simulink model "mod_sim_VTMS"  (R2018b)
settings: Solver=FixedStepDiscrete  StartTime=0.0  StopTime=t_Simulation  FixedStep=delta_t  RelTol=1e-3
values from neighbouring files (symbols this model uses):
  P_charge = 150    [main_sim_VTMS.m]
undefined symbols (not defined in the file or in its folder): A_EMaschine_Getriebe, A_j_c, A_Stirn, Anzahl_Peltierelemente, b_Batteriepack, b_c, b_EMaschine, b_Getriebe, b_j, b_Ladegeraet, BatPara, c_W, delta_t, DiscIntNeverNeededParam, e_Fahrzeug, eta_EMaschine_Break_M_EMaschine, eta_EMaschine_Break_n_EMaschine, eta_EMaschine_Faktor_Volllast, eta_EMaschine_Table, eta_Getriebe, eta_Ladegeraet, eta_Leistungselektronik_Break_M_EMaschine, eta_Leistungselektronik_Break_n_EMaschine, eta_Leistungselektronik_Faktor_Volllast, eta_Leistungselektronik_Table, f_R, I_DT_U_Break_DT, I_DT_U_Break_U, I_DT_U_Value_I, i_Getriebe, I_max, Ladevorgang, M_EMaschine_max, m_Fahrzeug, m_Zuladung, n_Zelle, P_Nebenverbraucher, p_Zelle, Peltier_Max_Eff, Q_DT_U_Break_DT, Q_DT_U_Break_U, Q_DT_U_Value_Q, Q_Imax_DT_Break_DT, Q_Imax_DT_Value_Q, r_dynamisch, rho_Luft, s_Zelle, SOC_init, Steuerung_Kuehlerluefter, Steuerung_Pumpe, Steuerung_Ventil, switch_BP_Zyklus, T_Batteriepack_init, T_EMaschine_Getriebe_init, T_Ladegeraet_init, T_Ladegeraet_Offset, T_Leistungselektronik_init, T_Offset_Batteriepack, T_Offset_EMaschine_Getriebe, T_Offset_Leistungselektronik ... (+36)
libraries: simulink x3, simulink_extras x2
(part 3 of 5)

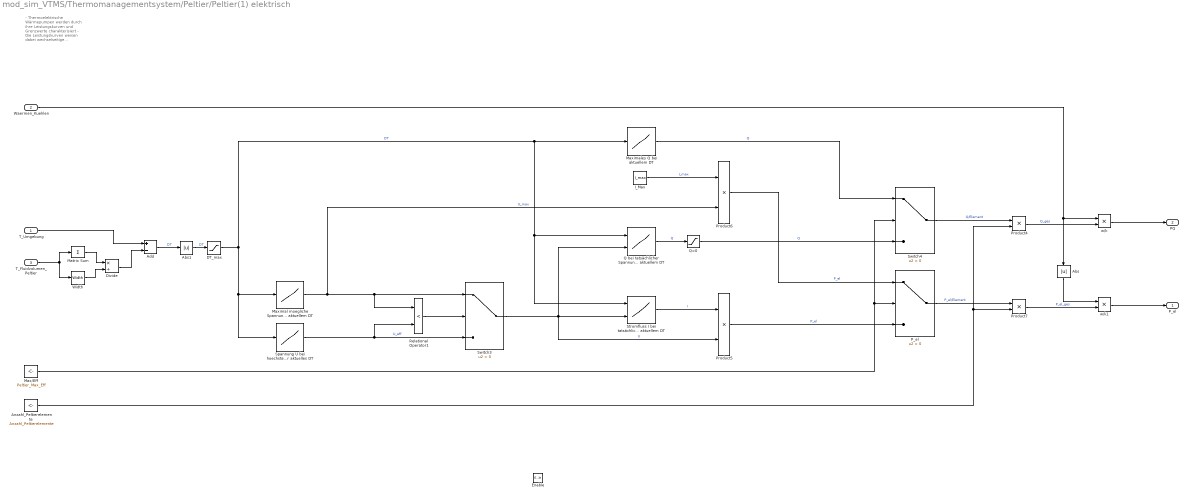
== system mod_sim_VTMS/Thermomanagementsystem/Peltier/Peltier(1) elektrisch ==
  note: - Thermoelektrische Wärmepumpen werden durch ihre Leistungskurven und Grenzwerte charakterisiert
      | - Die Leistungskurven weisen dabei wechselseitige Abhängigkeiten von der Temperaturdifferenz zwischen heißer und kalter Seite, der anliegenden Spannung, dem Strom und dem Wärmestrom auf.
      | - Für die Parameter existieren dabei Maximalwerte, die die Leistung und den Wärmefluss limitieren.
      | - Die Leistungskurven in diesem Modell sind aus dem Datenblatt einer beispielhaften Wärmepumpe entnommen.
      |
      | - Das Modell des Peltier-Elements hat keine eigene Masse und weist folglich keine eigene Temperatur auf
      | - Der resultierende Wärmestrom wird gesamthaft von einer Seite zur anderen transportiert, ohne dabei die Komponente aufzuheizen. Dadurch wirkt ein Wärmestrom direkt zwischen Umgebung und Kühlkreislauf und die Temperaturdifferenz zwischen heißer und kalter Seite ergibt sich aus der Umgebungstemperatur und der Temperatur des Kühlfluids
      | - Tendenziell ergibt sich für niedrigere Wärmeleistungen ein höherer COP. Deswegen wurden im Modell der Wärmepumpe zwei Betriebsmodi eingefügt, ein effektiver Modus und ein Leistungsmodus.
      | - Der Betriebsmodus wird über das Signal Max_Eff gesteuert, das den Wert 1 für maximale Leistung und den Wert -1 für maximale Effizienz annimmt.
      |
      | - Im effizienten Modus wird die Spannung an der Komponente so geregelt, dass sich für die aktuelle Temperaturdifferenz die höchste Leistungszahl ergibt. Das Maximum des COP liegt bei niedrigen Spannungen vor. Deswegen ergeben sich in diesem Zustand trotz der hohen Leistungszahl nur niedrige Wärmeleistungen.
      | - Im Leistungsmodus wird immer der maximal mögliche Wärmestrom erzeugt, ungeachtet vom COP. Dafür wird die Spannung so geregelt, dass sich entsprechend der aktuellen Temperaturdifferenz der maximale Strom einstellt, dieser aber nicht überschritten wird.
      |
      | Für detaillierte Informationen wird auf die schriftliche Arbeit von Bernhardt "Entwicklung und Auslegung eines innovativen Thermomanagementsystems für Elektrofahrzeuge" verwiesen.
  T_Umgebung : Inport
  Waermen_Kuehlen : Inport  Port=2
  T_Fluidvolumen_Peltier : Inport  Port=3
  Enable : EnablePort
  Abs : Abs
  Abs1 : Abs
  Add : Sum  Inputs=+-
  Anzahl_Peltierelemente : Constant  Value=Anzahl_Peltierelemente
  DT_max : Saturate  UpperLimit=60  LowerLimit=0
  Divide : Product  Inputs=*/
  I_Max : Constant  Value=I_max
  Matrix Sum : Sum  Inputs=+
  Max/Eff : Constant  Value=Peltier_Max_Eff
  Maximal moegliche Spannung bei aktuellem DT : Lookup_n-D  NumberOfTableDimensions=1  BreakpointsForDimension1=U_max_Break_DT  BreakpointsForDimension2=[1:3]  Table=U_max_Value_U  InternalRulePriority=Speed  RndMeth=Simplest  InputSameDT=on
  Maximales Q bei aktuellem DT : Lookup_n-D  NumberOfTableDimensions=1  BreakpointsForDimension1=Q_Imax_DT_Break_DT  BreakpointsForDimension2=[1:3]  Table=Q_Imax_DT_Value_Q  InternalRulePriority=Speed  RndMeth=Simplest  InputSameDT=on
  P_el : Switch  Criteria=u2 > Threshold
  Product{4..7} (4 alike) : Product
  Q bei tatsächlicher Spannung U und aktuellem DT : Lookup_n-D  BreakpointsForDimension1=Q_DT_U_Break_DT  BreakpointsForDimension2=Q_DT_U_Break_U  Table=Q_DT_U_Value_Q  InternalRulePriority=Speed  RndMeth=Simplest  InputSameDT=on
  Q>0 : Saturate  UpperLimit=inf  LowerLimit=0
  Relational Operator1 : RelationalOperator  Operator=<  OutDataTypeStr=boolean  RndMeth=Simplest
  Spannung U bei hoechsten COP fuer aktuelles DT : Lookup_n-D  NumberOfTableDimensions=1  BreakpointsForDimension1=U_COP_max_Break_DT  BreakpointsForDimension2=[1:3]  Table=U_COP_max_Value_U  InternalRulePriority=Speed  RndMeth=Simplest  InputSameDT=on
  Stromfluss I bei tatsächlicher Spannung U und aktuellem DT : Lookup_n-D  BreakpointsForDimension1=I_DT_U_Break_DT  BreakpointsForDimension2=I_DT_U_Break_U  Table=I_DT_U_Value_I  InternalRulePriority=Speed  RndMeth=Simplest  InputSameDT=on
  Switch3 : Switch  Criteria=u2 > Threshold
  Switch4 : Switch  Criteria=u2 > Threshold
  Width : Width
  w/k : Product
  w/k1 : Product
  "P_el " : Outport
  PQ : Outport  Port=2
  wires:
  Waermen_Kuehlen/1 -> Abs/1, w/k/1
  Relational Operator1/1 -> Switch3/2
  Q bei tatsächlicher Spannung U und aktuellem DT/1 -> Q>0/1  "Q"
  Maximal moegliche Spannung bei aktuellem DT/1 -> Product6/2, Switch3/1, Relational Operator1/1  "U_max"
  DT_max/1 -> Stromfluss I bei tatsächlicher Spannung U und aktuellem DT/1, Q bei tatsächlicher Spannung U und aktuellem DT/1, Maximales Q bei aktuellem DT/1, Spannung U bei hoechsten COP fuer aktuelles DT/1, Maximal moegliche Spannung bei aktuellem DT/1  "DT"
  Add/1 -> Abs1/1  "DT"
  Switch3/1 -> Q bei tatsächlicher Spannung U und aktuellem DT/2, Product5/2, Stromfluss I bei tatsächlicher Spannung U und aktuellem DT/2  "U"
  P_el/1 -> Product7/1  "P_el/Element"
  Product6/1 -> P_el/1  "P_el"
  I_Max/1 -> Product6/1  "I_max"
  Product4/1 -> w/k/2  "Q_ges"
  Spannung U bei hoechsten COP fuer aktuelles DT/1 -> Switch3/3, Relational Operator1/2  "U_eff"
  Max/Eff/1 -> Switch4/2, P_el/2
  Switch4/1 -> Product4/1  "Q/Element"
  w/k/1 -> PQ/1
  Stromfluss I bei tatsächlicher Spannung U und aktuellem DT/1 -> Product5/1  "I"
  Product5/1 -> P_el/3  "P_el"
  Anzahl_Peltierelemente/1 -> Product4/2, Product7/2
  Abs1/1 -> DT_max/1  "DT"
  Maximales Q bei aktuellem DT/1 -> Switch4/1  "Q"
  Product7/1 -> w/k1/2  "P_el_ges"
  Divide/1 -> Add/2
  Width/1 -> Divide/2
  T_Umgebung/1 -> Add/1
  Matrix Sum/1 -> Divide/1
  T_Fluidvolumen_Peltier/1 -> Matrix Sum/1, Width/1
  Q>0/1 -> Switch4/3  "Q"
  w/k1/1 -> "P_el "/1
  Abs/1 -> w/k1/1

== system mod_sim_VTMS/Thermomanagementsystem/Peltier/Peltier(1) thermisch ==
  note: -> Das Peltier-Element selber hat keine Masse
      | -> Es besitzt dadurch keine eigene Temperatur
      |
      | -> Es Transportiert die komplette Leistung als Wärme- oder Kühlleistung in das Kuehlwasser
      | -> Dafür wird die Leistung durch die Anzahl an finiten Volumen geteilt
      |
      | -> Die Peltier-Leistung wird in Form eines Vektors der Größe des Temperaturvektors, also der Anzahl an finiten Volumen in der Fluidkomponente, übertragen.
      | -> Dafür wird ein Einsvektor der Größe erstellt und mit der Leistung pro fintem Volumen multipliziert
  P_Peltier [W] : Inport
  T_FinitesVolumen [K] : Inport  Port=2
  Divide : Product  Inputs=*/
  Divide1 : Product  Inputs=*/
  Divide2 : Product  Inputs=**
  Width : Width
  PQ_Peltier_FinitesVolumen [W] : Outport
  wires:
  Width/1 -> Divide/2
  Divide1/1 -> Divide2/2
  Divide/1 -> Divide2/1
  T_FinitesVolumen [K]/1 -> Divide1/2, Divide1/1, Width/1
  Divide2/1 -> PQ_Peltier_FinitesVolumen [W]/1
  P_Peltier [W]/1 -> Divide/1  "P_Peltier [W]"

== system mod_sim_VTMS/Thermomanagementsystem/Rad_Betriebspunkt/Abbruch, wenn v_Fahrzeug > Schwellwert ==
  v_Fahrzeug [m/s] : Inport
  Enable : EnablePort
  Abbruchgeschwindigkeit [km/h] : Constant  Value=v_end
  Gain4 : Gain  Gain=3.6
  Relational Operator : RelationalOperator  OutDataTypeStr=boolean  RndMeth=Simplest
  Stop Simulation : Stop
  wires:
  Gain4/1 -> Relational Operator/1
  Abbruchgeschwindigkeit [km/h]/1 -> Relational Operator/2
  Relational Operator/1 -> Stop Simulation/1
  v_Fahrzeug [m/s]/1 -> Gain4/1

== system mod_sim_VTMS/Thermomanagementsystem/Schlauch/Schlauch thermisch ==
  note: -> Ein Schlauch besitzt keine eigene Temperatur und wird als adiabat zu seiner Umgebung betrachtet
      | -> Es gibt also keinen Wärmeaustausch zwischen Umgebungsluft und Kühlflüssigkeit
      | -> Ein Schlauch besitzt zudem nur 1 Strömungsgebiet bzw. 1 Kühlflüssigkeit
      | -> Deshalb existiert bei einem Schlauch kein Wärmeaustausch zwischen der Kühlflüssigkeit im Strömungsgebiet und ihrer Umgebung
      | -> Deswegen wird T_FinitesVolumen_i mit 0 multipliziert, um PQ_Schlauch_FinitesVolumen_i = 0 zu erhalten
      | -> Mit den unbenutzten Größen PV_Kuehlfluessigkeit und v_Fahrzeug (für die Wärmeübertragungsfähigkeit) sowie T_Umgebung und T_FinitesVolumen (für die Temperaturdifferenz zwischen Umgebungsluft und Kühlflüssigkeit) könnte aber ein Wärmeaustausch zwischen Umgebungsluft und Kühlflüssigkeit nachträglich modelliert werden, falls dies gewünscht sein sollte
  T_FinitesVolumen [K] : Inport
  PV_Kuehlfluessigkeit [m^3*s^-1] : Inport  Port=2
  T_Umgebung [K] : Inport  Port=3
  v_Fahrzeug [m*s^-1] : Inport  Port=4
  Gain : Gain  Gain=0
  Terminator : Terminator
  Terminator1 : Terminator
  Terminator2 : Terminator
  PQ_Schlauch_FinitesVolumen [W] : Outport
  wires:
  Gain/1 -> PQ_Schlauch_FinitesVolumen [W]/1
  PV_Kuehlfluessigkeit [m^3*s^-1]/1 -> Terminator/1
  v_Fahrzeug [m*s^-1]/1 -> Terminator2/1
  T_Umgebung [K]/1 -> Terminator1/1
  T_FinitesVolumen [K]/1 -> Gain/1

== system mod_sim_VTMS/Thermomanagementsystem/Wärmetauscher/Waermetauscher thermisch ==
  note: Gleichstromwärmetauscher (Art_Waermetauscher = 1):
      | PQ_Waermetauscher(1)_FinitesVolumen_i = UA_Waermetauscher_FinitesVolumen * (T_FinitesVolumen(2)_i - T_FinitesVolumen(1)_i) für i = 1:n
      | PQ_Waermetauscher(2)_FinitesVolumen_i = UA_Waermetauscher_FinitesVolumen * (T_FinitesVolumen(1)_i - T_FinitesVolumen(2)_i) für i = 1:n
      |
      | Gegenstromwärmetauscher (Art_Waermetauscher = -1):
      | PQ_Waermetauscher(1)_FinitesVolumen_i = UA_Waermetauscher_FinitesVolumen * (T_FinitesVolumen(2)_n+1-i - T_FinitesVolumen(1)_i) für i = 1:n
      | PQ_Waermetauscher(2)_FinitesVolumen_i = UA_Waermetauscher_FinitesVolumen * (T_FinitesVolumen(1)_n+1-i - T_FinitesVolumen(2)_i) für i = 1:n
      |
      | mit UA_Waermetauscher_FinitesVolumen = f (PV_Kuehlfluessigkeit(1), PV_Kuehlfluessigkeit(2))
      |
      | -> UA_Waermetauscher_FinitesVolumen ist für jedes finite Volumen des 1. bzw. 2. Strömungsgebiets eines Wärmetauschers identisch, weil das 1. bzw. 2. Strömungsgebiet eines Wärmetauschers durch identische finite Volumen örtlich diskretisiert ist und weil im gesamten 1. bzw. 2. Strömungsgebiet eines Wärmetauschers der gleiche Volumenstrom der Kühlflüssigkeit vorliegt
      | -> Im Thermomanagementsystemmodell geht der Massenstrom bzw. Volumenstrom innerhalb einer Fluid_Komponente bei jeder Fluid_Komponente stets vom 1. finiten Volumen zum n. finiten Volumen
      | -> Bei einem Gleichstromwärmetauscher sind die Kühlflüssigkeitsströme in seinen zwei Strömungsgebieten gleich gerichtet
      | -> Deswegen tauscht das i. finite Volumen des einen Strömungsgebiets des Wärmetauschers mit dem i. finiten Volumen des anderen Strömungsgebiets des Wärmetauschers Wärme aus
      | -> Bei einem Gegenstromwärmetauscher sind die Kühlflüssigkeitsströme in seinen zwei Strömungsgebieten entgegengesetzt gerichtet
      | -> Deswegen tauscht das i. finite Volumen des einen Strömungsgebiets des Wärmetauschers mit dem n+1-i. finiten Volumen des anderen Strömungsgebiets des Wärmetauschers Wärme aus
  note: -> Ein Wärmetauscher besitzt keine eigene Temperatur und wird als adiabat zu seiner Umgebung betrachtet
      | -> Es gibt also keinen Wärmeaustausch zwischen Umgebungsluft und Kühlflüssigkeit, sondern nur einen Wärmeaustausch zwischen den beiden Kühlflüssigkeiten eines Wärmetauschers
      | -> Mit den unbenutzten Größen T_Umgebung (für die Temperaturdifferenz zwischen Umgebungsluft und Kühlflüssigkeit) und v_Fahrzeug (für die Wärmeübertragungsfähigkeit) könnte aber ein Wärmeaustausch zwischen Umgebungsluft und Kühlflüssigkeit nachträglich modelliert werden, falls dies gewünscht sein sollte
  T_FinitesVolumen(1) [K] : Inport
  PV_Kuehlfluessigkeit(1) [m^3*s^-1] : Inport  Port=2
  T_FinitesVolumen(2) [K] : Inport  Port=3
  PV_Kuehlfluessigkeit(2) [m^3*s^-1] : Inport  Port=4
  T_Umgebung [K] : Inport  Port=5
  v_Fahrzeug [m*s^-1] : Inport  Port=6
  Art_Waermetauscher : Constant  Value=0  VectorParams1D=off
  Flip : DSPFlip
  Flip1 : DSPFlip
  Product : Product
  Product1 : Product
  Subtract : Sum  Inputs=+-
  Subtract1 : Sum  Inputs=+-
  Switch : Switch  Criteria=u2 > Threshold
  Switch1 : Switch  Criteria=u2 > Threshold
  Terminator : Terminator
  Terminator1 : Terminator
  n-D Lookup Table : Lookup_n-D  BreakpointsForDimension1=0  BreakpointsForDimension2=0  BreakpointsForDimension3=[5, 7]  BeginIndexSearchUsingPreviousIndexResult=on  Table=0  ExtrapMethod=Clip  UseLastTableValue=on  InternalRulePriority=Speed  RndMeth=Simplest  InputSameDT=on
  PQ_Waermetauscher(1)_FinitesVolumen [W] : Outport
  PQ_Waermetauscher(2)_FinitesVolumen [W] : Outport  Port=2
  wires:
  PV_Kuehlfluessigkeit(1) [m^3*s^-1]/1 -> n-D Lookup Table/1
  Subtract/1 -> Product/2
  n-D Lookup Table/1 -> Product/1, Product1/1  "UA_Waermetauscher_FinitesVolumen [W*K^-1]"
  Product/1 -> PQ_Waermetauscher(1)_FinitesVolumen [W]/1
  v_Fahrzeug [m*s^-1]/1 -> Terminator1/1
  T_Umgebung [K]/1 -> Terminator/1
  PV_Kuehlfluessigkeit(2) [m^3*s^-1]/1 -> n-D Lookup Table/2
  Flip/1 -> Switch/3
  Switch/1 -> Subtract/1
  T_FinitesVolumen(2) [K]/1 -> Switch/1, Flip/1, Subtract1/2
  Art_Waermetauscher/1 -> Switch/2, Switch1/2
  Subtract1/1 -> Product1/2
  Switch1/1 -> Subtract1/1
  Flip1/1 -> Switch1/3
  T_FinitesVolumen(1) [K]/1 -> Subtract/2, Switch1/1, Flip1/1
  Product1/1 -> PQ_Waermetauscher(2)_FinitesVolumen [W]/1

== system mod_sim_VTMS/Thermomanagementsystem/Batteriepack/Batteriepack(1) elektrisch/Batteriepackgrößen ==
  note: P_Verlust_Batteriepack = (P_Verlust_Zelle_irreversibel + P_Verlust_Zelle_reversibel) * n_Zelle
  note: U_Batteriepack = U_Zelle * s_Zelle
  note: I_Batteriepack = I_Zelle * p_Zelle
  note: -> Da alle Zellen als komplett identisch angenommen werden, entspricht der Wirkungsgrad einer Zelle dem Wirkungsgrad des gesamten Batteriepacks
      |
      | eta_Batteriepack = eta_Zelle
      | = P_Zelle / (P_Zelle + P_Verlust_Zelle_irreversibel) für P > 0
      | = (P_Zelle + P_Verlust_Zelle_irreversibel) / P_Zelle für P < 0
      |
      | -> Die Berechnung wird nur ausgeführt, wenn P_Zelle ~= 0 ist, weil bei P_Zelle = 0 auch P_Verlust_Zelle_irreversibel = 0 ist und dadurch eine Berechnung mit Division durch 0 durchgeführt werden würde (P_Zelle kann im Fahrbetrieb nicht < 0 sein, weil von den Rädern an den Antriebsstrang keine negativen Leistungsanforderungen übertragen werden)
      | -> Während der Batterieladung wird diese mit einem P < 0 geladen
      | -> Dies wird über das Subsystem "Enabled Subsystem" realisiert
      | -> Wenn P_Zelle = 0 ist, wird die Berechnung nicht durchgeführt und eta_Batteriepack solange auf dem gleichen Wert gehalten, bis P_Zelle wieder ~= 0 ist
  note: -> Der SOC des Batteriepacks entspricht dem SOC einer Zelle, weil alle Zellen im Batteriepack den gleichen Wert aufweisen
      |
      | SOC_Batteriepack = SOC_Zelle
  P_Zelle [W] : Inport
  I_Zelle [A] : Inport  Port=2
  U_Zelle [V] : Inport  Port=3
  SOC_Zelle [-] : Inport  Port=4
  P_Verlust_Zelle_irreversibel [W] : Inport  Port=5
  P_Verlust_Zelle_reversibel [W] : Inport  Port=6
  Abs : Abs
  Add : Sum
  Constant : Constant  Value=p_Zelle  VectorParams1D=off
  Constant1 : Constant  Value=s_Zelle  VectorParams1D=off
  Constant2 : Constant  Value=n_Zelle  VectorParams1D=off
  Enabled Subsystem : Subsystem  TreatAsAtomicUnit=on
  Product : Product
  Product1 : Product
  Product2 : Product
  I_Batteriepack [A] : Outport
  U_Batteriepack [V] : Outport  Port=2
  "SOC_Batteriepack [-] " : Outport  Port=3
  eta_Batteriepack [%] : Outport  Port=4
  P_Verlust_Batteriepack [W] : Outport  Port=5
  wires:
  Constant/1 -> Product/2
  I_Zelle [A]/1 -> Product/1
  Product/1 -> I_Batteriepack [A]/1
  U_Zelle [V]/1 -> Product1/1
  Constant1/1 -> Product1/2
  Product1/1 -> U_Batteriepack [V]/1
  Constant2/1 -> Product2/2
  Product2/1 -> P_Verlust_Batteriepack [W]/1
  Add/1 -> Product2/1
  P_Verlust_Zelle_reversibel [W]/1 -> Add/1
  SOC_Zelle [-]/1 -> "SOC_Batteriepack [-] "/1
  P_Verlust_Zelle_irreversibel [W]/1 -> Enabled Subsystem/1(P_Verlust_Zelle_irreversibel [W]), Add/2
  Enabled Subsystem/1(eta_Batteriepack [%]) -> eta_Batteriepack [%]/1
  Abs/1 -> Enabled Subsystem/Enable
  P_Zelle [W]/1 -> Abs/1, Enabled Subsystem/2(P_Zelle [W])

== system mod_sim_VTMS/Thermomanagementsystem/Batteriepack/Batteriepack(1) elektrisch/Zellmodell (abgeleitet aus Batteriepackmodell -> siehe FTM) ==
  I_Zelle [A] : Inport
  T_Zelle [°C] : Inport  Port=2
  Bus Creator2 : BusCreator  Inputs=4
  Bus Selector : BusSelector  OutputSignals=SOC
  Bus Selector1 : BusSelector  OutputSignals=SOC,U_Hysterese,U_RC1,U_RC2
  Ohmscher Spannungsanteil und Klemmenspannung der Zelle : Subsystem
  Potential der Zelle : Subsystem
  Unit Delay : UnitDelay  InitialCondition=SOC_init  SampleTime=-1
  Unit Delay1 : UnitDelay  InitialCondition=U_Hysterese_init  SampleTime=-1
  Unit Delay2 : UnitDelay  InitialCondition=U_RC1_init  SampleTime=-1
  Unit Delay3 : UnitDelay  InitialCondition=U_RC2_init  SampleTime=-1
  Unit Delay5 : UnitDelay  SampleTime=-1
  Unit Delay6 : UnitDelay  InitialCondition=T_Batteriepack_init-273.15  SampleTime=-1
  Verlustleistung der Zelle : Subsystem
  dt : Subsystem
  U_Zelle [V] : Outport
  SOC_Zelle [-] : Outport  Port=2
  P_Verlust_Zelle_irreversibel [W] : Outport  Port=3
  P_Verlust_Zelle_reversibel [W] : Outport  Port=4
  wires:
  Unit Delay3/1 -> Bus Creator2/4  "U_RC2"
  dt/1(dt [s]) -> Potential der Zelle/3(dt [s])
  Bus Selector1/3 -> Unit Delay2/1  "<U_RC1>"
  Unit Delay2/1 -> Bus Creator2/3  "U_RC1"
  Unit Delay6/1 -> Potential der Zelle/2(T_Zelle [°C])
  Unit Delay/1 -> Bus Creator2/1  "SOC"
  Bus Selector1/2 -> Unit Delay1/1  "<U_Hysterese>"
  Unit Delay1/1 -> Bus Creator2/2  "U_Hysterese"
  Bus Selector1/4 -> Unit Delay3/1  "<U_RC2>"
  Bus Creator2/1 -> Potential der Zelle/4(BatState_in)
  Bus Selector1/1 -> Unit Delay/1  "<SOC>"
  Potential der Zelle/2(BatPara) -> Ohmscher Spannungsanteil und Klemmenspannung der Zelle/3(BatPara), Verlustleistung der Zelle/4(BatPara)
  Potential der Zelle/1(U_Potential [V]) -> Ohmscher Spannungsanteil und Klemmenspannung der Zelle/2(U_Potential [V])
  Unit Delay5/1 -> Potential der Zelle/1(I_Zelle [A])
  Potential der Zelle/3(BatState_out) -> Bus Selector/1, Bus Selector1/1, Verlustleistung der Zelle/5(BatState)
  Ohmscher Spannungsanteil und Klemmenspannung der Zelle/2(U_Ohm [V]) -> Verlustleistung der Zelle/3(U_Ohm [V])
  T_Zelle [°C]/1 -> Unit Delay6/1, Verlustleistung der Zelle/1(T_Zelle [°C])
  I_Zelle [A]/1 -> Ohmscher Spannungsanteil und Klemmenspannung der Zelle/1(I_Zelle [A]), Verlustleistung der Zelle/2(I_Zelle [A]), Unit Delay5/1
  Verlustleistung der Zelle/1(P_Verlust_Zelle_irreversibel [W]) -> P_Verlust_Zelle_irreversibel [W]/1
  Ohmscher Spannungsanteil und Klemmenspannung der Zelle/1(U_Zelle [V]) -> U_Zelle [V]/1
  Verlustleistung der Zelle/2(P_Verlust_Zelle_reversibel [W]) -> P_Verlust_Zelle_reversibel [W]/1
  Bus Selector/1 -> SOC_Zelle [-]/1  "<SOC>"

== system mod_sim_VTMS/Thermomanagementsystem/Batteriepack/Batteriepack(1) thermisch/Waermeaustausch Batteriepack - Kuehlfluessigkeit ==
  note: PQ_Batteriepack_FinitesVolumen_i = UA_Batteriepack_FinitesVolumen * (T_Batteriepack - T_FinitesVolumen_i) für i = 1:n
      | PQ_Batteriepack_Kuehlfluessigkeit = Summe (PQ_Batteriepack_FinitesVolumen_i) für i = 1:n
      |
      | mit UA_Batteriepack_FinitesVolumen = f (PV_Kuehlfluessigkeit)
      |
      | -> UA_Batteriepack_FinitesVolumen ist für jedes finite Volumen des Strömungsgebiets des Batteriepacks identisch, weil das Strömungsgebiet des Batteriepacks durch identische finite Volumen örtlich diskretisiert ist und weil im gesamten Strömungsgebiet des Batteriepacks der gleiche Volumenstrom der Kühlflüssigkeit vorliegt
      | -> T_Batteriepack ist für jedes finite Volumen des Strömungsgebiets des Batteriepacks identisch, weil das Batteriepack als Blockkapazität aufgefasst wird
      | -> Der Wärmestrom zwischen dem Batteriepack und der gesamten Kühlflüssigkeit im Strömungsgebiet des Batteriepacks (wird für die thermische Modellierung des Batteriepacks benötigt) ergibt sich über die Summe aus den einzelnen Wärmeströmen zwischen dem Batteriepack und der Kühlflüssigkeit in einem finiten Volumen des Strömungsgebiets des Batteriepacks
  T_Batteriepack [K] : Inport
  T_FinitesVolumen [K] : Inport  Port=2
  PV_Kuehlfluessigkeit [m^3*s^-1] : Inport  Port=3
  1-D Lookup Table : Lookup_n-D  NumberOfTableDimensions=1  BreakpointsForDimension1=UA_Batteriepack_FinitesVolumen_Break_PV_Kuehlfluessigkeit{1}  BeginIndexSearchUsingPreviousIndexResult=on  Table=UA_Batteriepack_FinitesVolumen_Table{1}  ExtrapMethod=Clip  UseLastTableValue=on  InternalRulePriority=Speed  RndMeth=Simplest  InputSameDT=on
  Matrix Sum : Sum  Inputs=+
  Product : Product
  Subtract : Sum  Inputs=+-
  PQ_Batteriepack_Kuehlfluessigkeit [W] : Outport
  PQ_Batteriepack_FinitesVolumen [W] : Outport  Port=2
  wires:
  1-D Lookup Table/1 -> Product/1  "UA_Batteriepack_FinitesVolumen [W*K^-1]"
  T_Batteriepack [K]/1 -> Subtract/1
  Subtract/1 -> Product/2
  Matrix Sum/1 -> PQ_Batteriepack_Kuehlfluessigkeit [W]/1
  Product/1 -> PQ_Batteriepack_FinitesVolumen [W]/1, Matrix Sum/1
  PV_Kuehlfluessigkeit [m^3*s^-1]/1 -> 1-D Lookup Table/1
  T_FinitesVolumen [K]/1 -> Subtract/2

== system mod_sim_VTMS/Thermomanagementsystem/Batteriepack/Batteriepack(1) thermisch/Waermeaustausch Batteriepack - Umgebungsluft ==
  note: PQ_Batteriepack_Umgebung = UA_Batteriepack_Umgebung * (T_Batteriepack - T_Umgebung_Batteriepack)
      |
      | mit UA_Batteriepack_Umgebung = f (v_Fahrzeug)
      | mit T_Umgebung_Batteriepack = T_Umgebung + T_Offset_Batteriepack
      |
      | -> Durch T_Offset_Batteriepack ist die Temperatur der Umgebungsluft um das Batteriepack zur normalen Temperatur der Umgebungsluft verändert
  T_Batteriepack [K] : Inport
  T_Umgebung_Batteriepack [K] : Inport  Port=2
  v_Fahrzeug [m*s^-1] : Inport  Port=3
  1-D Lookup Table : Lookup_n-D  NumberOfTableDimensions=1  BreakpointsForDimension1=UA_Batteriepack_Umgebung_Break_v_Fahrzeug{1}  BeginIndexSearchUsingPreviousIndexResult=on  Table=UA_Batteriepack_Umgebung_Table{1}  ExtrapMethod=Clip  UseLastTableValue=on  InternalRulePriority=Speed  RndMeth=Simplest  InputSameDT=on
  Product1 : Product
  Subtract : Sum  Inputs=+-
  PQ_Batteriepack_Umgebung [W] : Outport
  wires:
  T_Batteriepack [K]/1 -> Subtract/1
  T_Umgebung_Batteriepack [K]/1 -> Subtract/2
  Product1/1 -> PQ_Batteriepack_Umgebung [W]/1
  1-D Lookup Table/1 -> Product1/1  "UA_Batteriepack_Umgebung [W*K^-1]"
  Subtract/1 -> Product1/2
  v_Fahrzeug [m*s^-1]/1 -> 1-D Lookup Table/1

== system mod_sim_VTMS/Thermomanagementsystem/E-Maschine/EMaschine(1) + Getriebe(1) thermisch/Waermeaustausch EMaschine - Kuehlfluessigkeit ==
  note: PQ_EMaschine_FinitesVolumen_i = UA_EMaschine_FinitesVolumen * (T_EMaschine - T_FinitesVolumen_i) für i = 1:n
      | PQ_EMaschine_Kuehlfluessigkeit = Summe (PQ_EMaschine_FinitesVolumen_i) für i = 1:n
      |
      | mit UA_EMaschine_FinitesVolumen = f (PV_Kuehlfluessigkeit)
      |
      | -> UA_EMaschine_FinitesVolumen ist für jedes finite Volumen des Strömungsgebiets der E-Maschine identisch, weil das Strömungsgebiet der E-Maschine durch identische finite Volumen örtlich diskretisiert ist und weil im gesamten Strömungsgebiet der E-Maschine der gleiche Volumenstrom der Kühlflüssigkeit vorliegt
      | -> T_EMaschine ist für jedes finite Volumen des Strömungsgebiets der E-Maschine identisch, weil die E-Maschine als Blockkapazität aufgefasst wird
      | -> Der Wärmestrom zwischen der E-Maschine und der gesamten Kühlflüssigkeit im Strömungsgebiet der E-Maschine (wird für die thermische Modellierung der E-Maschine benötigt) ergibt sich über die Summe aus den einzelnen Wärmeströmen zwischen der E-Maschine und der Kühlflüssigkeit in einem finiten Volumen des Strömungsgebiets der E-Maschine
  T_EMaschine [K] : Inport
  T_FinitesVolumen [K] : Inport  Port=2
  PV_Kuehlfluessigkeit [m^3*s^-1] : Inport  Port=3
  1-D Lookup Table : Lookup_n-D  NumberOfTableDimensions=1  BreakpointsForDimension1=UA_EMaschine_FinitesVolumen_Break_PV_Kuehlfluessigkeit{1}  BeginIndexSearchUsingPreviousIndexResult=on  Table=UA_EMaschine_FinitesVolumen_Table{1}  ExtrapMethod=Clip  UseLastTableValue=on  InternalRulePriority=Speed  RndMeth=Simplest  InputSameDT=on
  Matrix Sum : Sum  Inputs=+
  Product : Product
  Subtract : Sum  Inputs=+-
  PQ_EMaschine_Kuehlfluessigkeit [W] : Outport
  PQ_EMaschine_FinitesVolumen [W] : Outport  Port=2
  wires:
  1-D Lookup Table/1 -> Product/1  "UA_EMaschine_FinitesVolumen [W*K^-1]"
  T_EMaschine [K]/1 -> Subtract/1
  Subtract/1 -> Product/2
  Matrix Sum/1 -> PQ_EMaschine_Kuehlfluessigkeit [W]/1
  Product/1 -> PQ_EMaschine_FinitesVolumen [W]/1, Matrix Sum/1
  PV_Kuehlfluessigkeit [m^3*s^-1]/1 -> 1-D Lookup Table/1
  T_FinitesVolumen [K]/1 -> Subtract/2

== system mod_sim_VTMS/Thermomanagementsystem/E-Maschine/EMaschine(1) + Getriebe(1) thermisch/Waermeaustausch EMaschine - Umgebungsluft  ==
  note: PQ_EMaschine_Umgebung = UA_EMaschine_Umgebung * (T_EMaschine - T_Umgebung_EMaschine_Getriebe)
      |
      | mit UA_EMaschine_Umgebung = f (v_Fahrzeug)
      | mit T_Umgebung_EMaschine_Getriebe = T_Umgebung + T_Offset_EMaschine_Getriebe
      |
      | -> Durch T_Offset_EMaschine_Getriebe ist die Temperatur der Umgebungsluft um die E-Maschine zur normalen Temperatur der Umgebungsluft verändert
  T_EMaschine [K] : Inport
  T_Umgebung_EMaschine_Getriebe [K] : Inport  Port=2
  v_Fahrzeug [m*s^-1] : Inport  Port=3
  1-D Lookup Table : Lookup_n-D  NumberOfTableDimensions=1  BreakpointsForDimension1=UA_EMaschine_Umgebung_Break_v_Fahrzeug{1}  BeginIndexSearchUsingPreviousIndexResult=on  Table=UA_EMaschine_Umgebung_Table{1}  ExtrapMethod=Clip  UseLastTableValue=on  InternalRulePriority=Speed  RndMeth=Simplest  InputSameDT=on
  Product : Product
  Subtract : Sum  Inputs=+-
  PQ_EMaschine_Umgebung [W] : Outport
  wires:
  T_EMaschine [K]/1 -> Subtract/1
  T_Umgebung_EMaschine_Getriebe [K]/1 -> Subtract/2
  Product/1 -> PQ_EMaschine_Umgebung [W]/1
  1-D Lookup Table/1 -> Product/1  "UA_EMaschine_Umgebung [W*K^-1]"
  Subtract/1 -> Product/2
  v_Fahrzeug [m*s^-1]/1 -> 1-D Lookup Table/1

== system mod_sim_VTMS/Thermomanagementsystem/E-Maschine/EMaschine(1) + Getriebe(1) thermisch/Waermeaustausch Getriebe - Umgebungsluft ==
  note: PQ_Getriebe_Umgebung = UA_Getriebe_Umgebung * (T_Getriebe - T_Umgebung_EMaschine_Getriebe)
      |
      | mit UA_Getriebe_Umgebung = f (v_Fahrzeug)
      | mit T_Umgebung_EMaschine_Getriebe = T_Umgebung + T_Offset_EMaschine_Getriebe
      |
      | -> Durch T_Offset_EMaschine_Getriebe ist die Temperatur der Umgebungsluft um das Getriebe  zur normalen Temperatur der Umgebungsluft verändert
  T_Getriebe [K] : Inport
  T_Umgebung_EMaschine_Getriebe [K] : Inport  Port=2
  v_Fahrzeug [m*s^-1] : Inport  Port=3
  1-D Lookup Table : Lookup_n-D  NumberOfTableDimensions=1  BreakpointsForDimension1=UA_Getriebe_Umgebung_Break_v_Fahrzeug{1}  BeginIndexSearchUsingPreviousIndexResult=on  Table=UA_Getriebe_Umgebung_Table{1}  ExtrapMethod=Clip  UseLastTableValue=on  InternalRulePriority=Speed  RndMeth=Simplest  InputSameDT=on
  Product2 : Product
  Subtract : Sum  Inputs=+-
  PQ_Getriebe_Umgebung [W] : Outport
  wires:
  T_Getriebe [K]/1 -> Subtract/1
  T_Umgebung_EMaschine_Getriebe [K]/1 -> Subtract/2
  Subtract/1 -> Product2/2
  Product2/1 -> PQ_Getriebe_Umgebung [W]/1
  1-D Lookup Table/1 -> Product2/1  "UA_Getriebe_Umgebung [W*K^-1]"
  v_Fahrzeug [m*s^-1]/1 -> 1-D Lookup Table/1

== system mod_sim_VTMS/Thermomanagementsystem/Fluid/Bestimmung PV_Kuehlkreislauf/Kuehlkreislauf ==
  note: -> Eine Pumpe wird nicht modelliert
      | -> Es wird nur der Volumenstrom im Kühlkreislauf, für den eine Pumpe sorgt, benötigt
      | -> Pumpen gesteuert (Steuerung_Pumpe = 1): PV_Kuehlkreislauf wird über Steuerung in Subsystem "Steuerung Pumpe" bestimmt
      | -> Pumpen ungesteuert (Steuerung_Pumpe = 0): PV_Kuehlkreislauf wird zeitabhängig vom Anwender vorgegeben
  note: -> Ein Kühlkreislauf besitzt eine Pumpe, die für den Volumenstrom im Kühlkreislauf sorgt
      | -> Eine Pumpe wird als 0D angenommen
      | -> Je nachdem wie es der Anwender wünscht, können Pumpen gesteuert oder ungesteuert sein
  EMaschine_Output : Inport
  Leistungselektronik_Output : Inport  Port=2
  Batteriepack_Output : Inport  Port=3
  Constant : Constant  Value=Steuerung_Pumpe  VectorParams1D=off
  PV_Kuehlkreislauf : FromWorkspace  VariableName=[0 0]  SampleTime=0
  Steuerung Pumpe : Subsystem
  Switch : Switch  Criteria=u2 > Threshold
  PV_Kuehlkreislauf [m^3*s^-1] : Outport
  wires:
  Steuerung Pumpe/1(PV_Kuehlkreislauf [m^3*s^-1]) -> Switch/1
  Constant/1 -> Switch/2
  PV_Kuehlkreislauf/1 -> Switch/3
  EMaschine_Output/1 -> Steuerung Pumpe/1(EMaschine_Output)
  Switch/1 -> PV_Kuehlkreislauf [m^3*s^-1]/1
  Leistungselektronik_Output/1 -> Steuerung Pumpe/2(Leistungselektronik_Output)
  Batteriepack_Output/1 -> Steuerung Pumpe/3(Batteriepack_Output)

== system mod_sim_VTMS/Thermomanagementsystem/Fluid/Bestimmung Zustand_Ventil/Ventil ==
  note: -> In einem Kühlkreislauf können Dreiwegeventile sein
      | -> Ein Dreiwegeventil wird als 0D angenommen
      | -> Je nachdem wie es der Anwender wünscht, können Dreiwegeventile gesteuert oder ungesteuert sein
  note: -> Ein Dreiwegeventil wird nicht modelliert
      | -> Es wird der Zustand eines Dreiwegeventils benötigt
      | -> Dreiwegeventile gesteuert (Steuerung_Ventil = 1): Zustand_Ventil wird über Steuerung in Subsystem "Steuerung Ventil" bestimmt
      | -> Dreiwegeventile ungesteuert (Steuerung_Ventil = 0): Zustand_Ventil wird zeitabhängig vom Anwender vorgegeben
      |
      | -> Im Thermomanagementsystemmodell werden Berechnungen mit Divison durch Zustand_Ventil bzw. 1-Zustand_Ventil durchgeführt
      | -> Da eine Berechnung mit Division durch 0 nicht möglich ist, wird Zustand_Ventil immer zwischen 0.001 und 0.999 skaliert (Block "Saturation")
      | -> Damit gibt es keinen Rechenfehler bzw. die Simulation ist stabil, aber es ist immer (auch bei offiziellen Zustand_Ventil = 0 oder 1) zumindest ein minimaler Volumenstrom der Kühlflüssigkeit im Neben- bzw. Hauptpfad eines Dreiwegeventils vorhanden
      | -> Folglich wird für das Thermomanagementsystemmodell angenommen, dass ein Dreiwegeventil nicht komplett abdichten kann
      | -> Dies kann dadurch validiert werden, dass ein Dreiwegeventil in der Realität in der Regel auch nicht komplett abdichtet
  Fluid_Schlauch_Output : Inport
  Constant : Constant  Value=Steuerung_Ventil  VectorParams1D=off
  Saturation : Saturate  UpperLimit=0.999  LowerLimit=0.001
  Steuerung Ventil : Subsystem
  Switch : Switch  Criteria=u2 > Threshold
  Zustand_Ventil : FromWorkspace  VariableName=[0 0]  SampleTime=0
  Zustand_Ventil [-] : Outport
  wires:
  Switch/1 -> Saturation/1
  Fluid_Schlauch_Output/1 -> Steuerung Ventil/1(Fluid_Schlauch_Output)
  Zustand_Ventil/1 -> Switch/3
  Constant/1 -> Switch/2
  Steuerung Ventil/1(Zustand_Ventil [-]) -> Switch/1
  Saturation/1 -> Zustand_Ventil [-]/1

== system mod_sim_VTMS/Thermomanagementsystem/Fluid/Fluid_Komponente thermisch/Bestimmung PV_Kuehlfluessigkeit ==
  note: -> Ein finites Volumen ist stets vollständig mit Kühlflüssigkeit gefüllt
      | -> Deswegen gilt für ein finites Volumen die Massenerhaltung -> Eintretender Massenstrom und austretender Massenstrom sind identisch
      | -> Wegen der Annahme, dass die Kühflüssigkeit in einem Kühlkreislauf ein inkommpressibles Fluid ist, und weil ein homogenes Dichtefeld in einem Kühlkreislauf angenommen wird, gilt für ein finites Volumen ebenso die Volumenerhaltung -> Eintretender Volumenstrom und austretender Volumenstrom sind identisch
      | -> Zusätzlich gilt innerhalb einer Fluid_Komponente an der Grenzfläche zwischen finite Volumen, dass der austretende Volumenstrom aus dem vorherigen finiten Volumen und der eintretende Volumenstrom in das nachfolgende finte Volumen identisch ist
      | -> Deswegen liegt in einer Fluid_Komponente der gleiche Volumenstrom vor
      | -> Ein Dreiwegeventil befindet sich zwischen Fluid_Komponenten, wird aber als 0D angenommen
      | -> Der Volumenstrom vor einem Dreiwegeventil (in der vorherigen Fluid_Komponente bzw. im vorherigen finiten Volumen) teilt sich nach dem Dreiwegeventil auf die beiden Pfade (Hauptpfad und Nebenpfad) des Dreiwegeventils (auf zwei nachkommende Fluid_Komponenten bzw. auf zwei nachkommende finite Volumen) auf
      | -> Dies geschieht entsprechend dem Zustand des Dreiwegeventils
      | -> Hauptpfad: 1-Zustand_Ventil; Nebenpfad: Zustand_Ventil
      | -> Hauptpfad: Bei Zustand_Ventil = 0 fließt alles über den Hauptpfad, bei Zustand_Ventil = 1 fließt nichts über den Hauptpfad
      | -> Nebenpfad: Bei Zustand_Ventil = 0 fließt nichts über den Nebenpfad, bei Zustand_Ventil = 1 fließt alles über den Nebenpfad
      | -> Der Anwender legt in MATLAB fest, in welchem Pfad des Dreiwegeventils sich eine Fluid_Komponente befindet
      | -> PV_Kuehlkreislauf_Faktor_Ventil entspricht dann einem dieser Zustände des entsprechenden Dreiwegeventils, je nachdem, ob sich die Fluid_Komponente innerhalb des Hauptpfades (PV_Kuehlkreislauf_Faktor_Ventil = 1-Zustand_Ventil) oder innerhalb des Nebenpfades (PV_Kuehlkreislauf_Faktor_Ventil = Zustand_Ventil) des entsprechenden Dreiwegeventils befindet
  note: -> PV_Kuehlkreislauf ist der Volumenstrom in dem entsprechenden Kühlkreislauf, in dem sich die Fluid_Komponente befindet
      | -> Wenn sich die Fluid_Komponente innerhalb von Pfaden von Dreiwegeventilen befindet, ist der Volumenstrom der Kühlflüssgkeit in der Fluid_Komponente zusätzlich zu PV_Kuehlkreislauf abh. von den Zuständen dieser Dreiwegeventile und in welchen Pfaden (Hauptpfad oder Nebenpfad) der Dreiwegeventile sich die Fluid_Komponente befindet
      | -> Dies wird über die Multiplikation von PV_Kuehlkreislauf mit PV_Kuehlkreislauf_Faktor_gesamt berücksichtigt
      | -> Dadurch ergibt sich der korrekte Volumenstrom der Kühlflüssigkeit in der Fluid_Komponente
      |
      | PV_Kuehlfluessigkeit = PV_Kuehlkreislauf * PV_Kuehlkreislauf_Faktor_gesamt
      |
      | mit PV_Kuehlkreislauf_Faktor_gesamt, falls sich die Fluid_Komponente innerhalb Dreiwegeventil/e befindet:
      | PV_Kuehlkreislauf_Faktor_gesamt = 1 * Product (PV_Kuehlkreislauf_Faktor_Ventil(i)) für i = Nummer all derer Dreiwegeventile, innerhalb derer sich die Fluid_Komponente befindet
      |
      | mit PV_Kuehlkreislauf_Faktor_gesamt, falls sich die Fluid_Komponente NICHT innerhalb Dreiwegeventil/e befindet:
      | PV_Kuehlkreislauf_Faktor_gesamt = 1
      | -> PV_Kuehlfluessigkeit = PV_Kuehlkreislauf
      | -> In der Fluid_Komponente fließt dann PV_Kuehlkreislauf
  PV_Kuehlkreislauf [m^3*s^-1] : Inport
  Zustand_Ventil [-] : Inport  Port=2
  Constant : Constant  VectorParams1D=off
  Product : Product  Inputs=1
  Product1 : Product
  Ventil : Subsystem
  PV_Kuehlfluessigkeit [m^3*s^-1] : Outport
  wires:
  Product1/1 -> PV_Kuehlfluessigkeit [m^3*s^-1]/1
  PV_Kuehlkreislauf [m^3*s^-1]/1 -> Product1/1
  Product/1 -> Product1/2  "PV_Kuehlkreislauf_Faktor_gesamt [-]"
  Constant/1 -> Product/1

== system mod_sim_VTMS/Thermomanagementsystem/Fluid/Fluid_Komponente thermisch/Energiestroeme 1. finites Volumen durch Kopplung mit vorherigen Fluid_Komponenten - Vereinigung ==
  note: delta_PE_FinitesVolumen_1 = rho_Kuehlfluessigkeit * c_Kuehlfluessigkeit * (PV_FinitesVolumen_vor1 * T_FinitesVolumen_vor1_n + PV_FinitesVolumen_vor2 * T_FinitesVolumen_vor2_n - PV_FinitesVolumen * T_FinitesVolumen_1)
      | = rho_Kuehlfluessigkeit * c_Kuehlfluessigkeit * (PV_Kuehlfluessigkeit_vor1 * T_FinitesVolumen_vor1_n + PV_Kuehlfluessigkeit_vor2 * T_FinitesVolumen_vor2_n - PV_Kuehlfluessigkeit * T_FinitesVolumen_1)
      | = Differenz der Energieströme zwischen Eingang und Ausgang des 1. finiten Volumens
      |
      | -> Dieses Subsystem repäsentiert den Fall, dass sich diese Fluid_Komponente nach 2 Fluid_Komponenten befindet
      | -> Diese Fluid_Komponente befindet sich nach der Vereinigung der zwei nach der Aufzweigung durch ein Dreiwegeventil resultierenden Pfade
      | -> Deswegen gibt es zwei eintretende Massenströme bzw. Volumenströme
      |
      | -> Innerhalb einer Fluid_Komponente gilt für die gesamte Kühlflüssigkeit und damit für jedes und auch für das 1. finite Volumen: rho_Kuehlfluessigkeit = const., c_Kuehlfluessigkeit = const., weil ein homogenes Dichtefeld sowie ein örtlich konstanter Druck angenommen wird und die spezische Wärmekapazität temperaturunabhängig betrachtet wird
      | -> Der in ein finites Volumen eintretende Volumenstrom der Kühlflüssigkeit ist gleich dem aus diesem finiten Volumen austretenden Volumenstrom der Kühlflüssigkeit (-> siehe Subsystem "Bestimmung PV_Kuehlfluessigkeit" für Erklärung)
      | -> PV_FinitesVolumen = Ein- bzw. austretender Volumenstrom der Kühlflüssigkeit bzgl. eines finiten Volumens
      | -> Da PV_FinitesVolumen für jedes finite Volumen einer Fluid_Komponente identisch ist, liegt in einer Fluid_Komponente der gleiche Volumenstrom vor
      | -> Deswegen gilt: PV_FinitesVolumen = PV_Kuehlfluessigkeit
      | -> Für die Differenz der Energieströme zwischen Eingang und Ausgang des 1. finiten Volumens werden die Temperaturen der Kühlflüssigkeit am Eingang und Ausgang benötigt
      | -> Diese werden über die Temperaturen der Kühlflüssigkeit bzgl. der Knoten der finiten Volumen interpoliert
      | -> Als Interpolationsschema wird die Aufwind-Interpolation verwendet
      | -> Daraus folgt für diesen Fall für das 1. finite Volumen: Temperatur der Kühlflüssigkeit am Eingang = T_FinitesVolumen_vor1_n bzw. T_FinitesVolumen_vor2_n, weil es zwei eintretende Massenströme bzw. Volumenströme von zwei Fluid_Komponenten gibt (PV_Kuehlfluessigkeit_vor1 bzw. PV_Kuehlfluessigkeit_vor2 -> PV_Kuehlfluessigkeit = PV_Kuehlfluessigkeit_vor1 + PV_Kuehlfluessigkeit_vor2); Temperatur der Kühlflüssigkeit am Ausgang = T_FinitesVolumen_1
      | -> Wegen der zwei eintretenden Massenströme bzw. Volumenströme mit jeweils einer eigenen Temperatur der Kühlflüssigkeit am Eingang ergeben sich zwei verschiedene eintretende Energieströme
      | -> Da es sich bei Energieströmen um Leistungen handelt und Leistungen addiert werden können, ergibt sich der gesamte Energiestrom am Eingang über die Summe der beiden einzelnen Energieströme
      | -> Dadurch ergibt sich für diesen Fall für die Differenz der Energieströme zwischen Eingang und Ausgang des 1. finiten Volumens die obige Formel
      |
      | -> Für die Herleitung dieses mathematischen Zusammenhangs wird auf die auf die im Rahmen des Thermomanagementsystemmodells erstellte Masterarbeit "Entwicklung und Steuerung eines Thermomanagementsystemmodells für Elektrofahrzeuge" verwiesen
  T_FinitesVolumen [K] : Inport
  PV_Kuehlfluessigkeit [m^3*s^-1] : Inport  Port=2
  rho_Kuehlfluessigkeit [kg*m^-3] : Inport  Port=3
  c_Kuehlfluessigkeit [J*kg^-1*K^-1] : Inport  Port=4
  T_FinitesVolumen_vor1 [K] : Inport  Port=5
  PV_Kuehlfluessigkeit_vor1 [m^3*s^-1] : Inport  Port=6
  T_FinitesVolumen_vor2 [K] : Inport  Port=7
  PV_Kuehlfluessigkeit_vor2 [m^3*s^-1] : Inport  Port=8
  MATLAB Function : MATLAB Function  TreatAsAtomicUnit=on
  Product : Product
  delta_PE_FinitesVolumen [W] : Outport
  wires:
  MATLAB Function/1(y) -> delta_PE_FinitesVolumen [W]/1
  T_FinitesVolumen [K]/1 -> MATLAB Function/1(u)
  T_FinitesVolumen_vor1 [K]/1 -> MATLAB Function/2(v)
  T_FinitesVolumen_vor2 [K]/1 -> MATLAB Function/3(w)
  Product/1 -> MATLAB Function/4(a)
  PV_Kuehlfluessigkeit [m^3*s^-1]/1 -> MATLAB Function/5(b)
  rho_Kuehlfluessigkeit [kg*m^-3]/1 -> Product/1
  c_Kuehlfluessigkeit [J*kg^-1*K^-1]/1 -> Product/2
  PV_Kuehlfluessigkeit_vor1 [m^3*s^-1]/1 -> MATLAB Function/6(c)
  PV_Kuehlfluessigkeit_vor2 [m^3*s^-1]/1 -> MATLAB Function/7(d)

== system mod_sim_VTMS/Thermomanagementsystem/Fluid/Fluid_Komponente thermisch/Energiestroeme 1. finites Volumen durch Kopplung mit vorheriger Fluid_Komponente - normal+Ventil ==
  note: delta_PE_FinitesVolumen_1 = rho_Kuehlfluessigkeit * c_Kuehlfluessigkeit * PV_FinitesVolumen * (T_FinitesVolumen_vor1_n - T_FinitesVolumen_1)
      | = rho_Kuehlfluessigkeit * c_Kuehlfluessigkeit * PV_Kuehlfluessigkeit * (T_FinitesVolumen_vor1_n - T_FinitesVolumen_1)
      | = Differenz der Energieströme zwischen Eingang und Ausgang des 1. finiten Volumens
      |
      | -> Dieses Subsystem repräsentiert den Fall, dass sich diese Fluid_Komponente nach 1 Fluid_Komponente befindet
      | -> Es ist irrelevant, ob sich zwischen den beiden Fluid_Komponenten ein Dreiwegeventil befindet oder nicht
      | -> Deswegen gibt es nur einen eintretenden Massenstrom bzw. Volumenstrom
      |
      | -> Innerhalb einer Fluid_Komponente gilt für die gesamte Kühlflüssigkeit und damit für jedes und auch für das 1. finite Volumen: rho_Kuehlfluessigkeit = const., c_Kuehlfluessigkeit = const., weil ein homogenes Dichtefeld sowie ein örtlich konstanter Druck angenommen wird und die spezische Wärmekapazität temperaturunabhängig betrachtet wird
      | -> Der in ein finites Volumen eintretende Volumenstrom der Kühlflüssigkeit ist gleich dem aus diesem finiten Volumen austretenden Volumenstrom der Kühlflüssigkeit (-> siehe Subsystem "Bestimmung PV_Kuehlfluessigkeit" für Erklärung)
      | -> PV_FinitesVolumen = Ein- bzw. austretender Volumenstrom der Kühlflüssigkeit bzgl. eines finiten Volumens
      | -> Da PV_FinitesVolumen für jedes finite Volumen einer Fluid_Komponente identisch ist, liegt in einer Fluid_Komponente der gleiche Volumenstrom vor
      | -> Deswegen gilt: PV_FinitesVolumen = PV_Kuehlfluessigkeit
      | -> Für die Differenz der Energieströme zwischen Eingang und Ausgang des 1. finiten Volumens werden die Temperaturen der Kühlflüssigkeit am Eingang und Ausgang benötigt
      | -> Diese werden über die Temperaturen der Kühlflüssigkeit bzgl. der Knoten der finiten Volumen interpoliert
      | -> Als Interpolationsschema wird die Aufwind-Interpolation verwendet
      | -> Daraus folgt für diesen Fall für das 1. finite Volumen: Temperatur der Kühlflüssigkeit am Eingang = T_FinitesVolumen_vor1_n; Temperatur der Kühlflüssigkeit am Ausgang = T_FinitesVolumen_1
      |
      | -> Für die Herleitung dieses mathematischen Zusammenhangs wird auf die auf die im Rahmen des Thermomanagementsystemmodells erstellte Masterarbeit "Entwicklung und Steuerung eines Thermomanagementsystemmodells für Elektrofahrzeuge" verwiesen
  T_FinitesVolumen [K] : Inport
  PV_Kuehlfluessigkeit [m^3*s^-1] : Inport  Port=2
  rho_Kuehlfluessigkeit [kg*m^-3] : Inport  Port=3
  c_Kuehlfluessigkeit [J*kg^-1*K^-1] : Inport  Port=4
  T_FinitesVolumen_vor1 [K] : Inport  Port=5
  MATLAB Function : MATLAB Function  TreatAsAtomicUnit=on
  Product : Product  Inputs=3
  delta_PE_FinitesVolumen [W] : Outport
  wires:
  MATLAB Function/1(y) -> delta_PE_FinitesVolumen [W]/1
  T_FinitesVolumen [K]/1 -> MATLAB Function/1(u)
  T_FinitesVolumen_vor1 [K]/1 -> MATLAB Function/2(v)
  c_Kuehlfluessigkeit [J*kg^-1*K^-1]/1 -> Product/3
  PV_Kuehlfluessigkeit [m^3*s^-1]/1 -> Product/1
  rho_Kuehlfluessigkeit [kg*m^-3]/1 -> Product/2
  Product/1 -> MATLAB Function/3(a)

== system mod_sim_VTMS/Thermomanagementsystem/Fluid/Fluid_Komponente thermisch/Energiestroeme finite Volumen innerhalb Fluid_Komponente ==
  note: delta_PE_FinitesVolumen_i = rho_Kuehlfluessigkeit * c_Kuehlfluessigkeit * PV_FinitesVolumen * (T_FinitesVolumen_i-1 - T_FinitesVolumen_i) für i = 2 ... n
      | = rho_Kuehlfluessigkeit * c_Kuehlfluessigkeit * PV_Kuehlfluessigkeit * (T_FinitesVolumen_i-1 - T_FinitesVolumen_i) für i = 2 ... n
      | = Differenz der Energieströme zwischen Eingang und Ausgang des i. finiten Volumens für i = 2 ... n
      |
      | -> Innerhalb einer Fluid_Komponente gilt für die gesamte Kühlflüssigkeit und damit für jedes finite Volumen: rho_Kuehlfluessigkeit = const., c_Kuehlfluessigkeit = const., weil ein homogenes Dichtefeld sowie ein örtlich konstanter Druck angenommen wird und die spezische Wärmekapazität temperaturunabhängig betrachtet wird
      | -> Der in ein finites Volumen eintretende Volumenstrom der Kühlflüssigkeit ist gleich dem aus diesem finiten Volumen austretenden Volumenstrom der Kühlflüssigkeit (-> siehe Subsystem "Bestimmung PV_Kuehlfluessigkeit" für Erklärung)
      | -> PV_FinitesVolumen = Ein- bzw. austretender Volumenstrom der Kühlflüssigkeit bzgl. eines finiten Volumens
      | -> Da PV_FinitesVolumen für jedes finite Volumen einer Fluid_Komponente identisch ist, liegt in einer Fluid_Komponente der gleiche Volumenstrom vor
      | -> Deswegen gilt: PV_FinitesVolumen = PV_Kuehlfluessigkeit
      | -> Für die Differenz der Energieströme zwischen Eingang und Ausgang eines finiten Volumens werden für jedes finite Volumen die Temperaturen der Kühlflüssigkeit am Eingang und Ausgang benötigt
      | -> Diese werden über die Temperaturen der Kühlflüssigkeit bzgl. der Knoten der finiten Volumen interpoliert
      | -> Als Interpolationsschema wird die Aufwind-Interpolation verwendet
      | -> Daraus folgt für das i. finite Volumen: Temperatur der Kühlflüssigkeit am Eingang = T_FinitesVolumen_i-1; Temperatur der Kühlflüssigkeit am Ausgang = T_FinitesVolumen_i
      | -> Deshalb ist die Bestimmung der Differenz der Energieströme zwischen Eingang und Ausgang eines finiten Volumens innerhalb einer Fluid_Komponente nur für i = 2 ... n möglich
      | -> Die Bestimmung der Differenz der Energieströme zwischen Eingang und Ausgang des 1. finiten Volumens wird durch die Kopplungsfälle dargestellt
      |
      | -> Für die Herleitung dieses mathematischen Zusammenhangs wird auf die auf die im Rahmen des Thermomanagementsystemmodells erstellte Masterarbeit "Entwicklung und Steuerung eines Thermomanagementsystemmodells für Elektrofahrzeuge" verwiesen
  T_FinitesVolumen [K] : Inport
  PV_Kuehlfluessigkeit [m^3*s^-1] : Inport  Port=2
  rho_Kuehlfluessigkeit [kg*m^-3] : Inport  Port=3
  c_Kuehlfluessigkeit [J*kg^-1*K^-1] : Inport  Port=4
  MATLAB Function : MATLAB Function  TreatAsAtomicUnit=on
  Product : Product  Inputs=3
  delta_PE_FinitesVolumen [W] : Outport
  wires:
  MATLAB Function/1(y) -> delta_PE_FinitesVolumen [W]/1
  T_FinitesVolumen [K]/1 -> MATLAB Function/1(u)
  PV_Kuehlfluessigkeit [m^3*s^-1]/1 -> Product/1
  rho_Kuehlfluessigkeit [kg*m^-3]/1 -> Product/2
  c_Kuehlfluessigkeit [J*kg^-1*K^-1]/1 -> Product/3
  Product/1 -> MATLAB Function/2(a)

== system mod_sim_VTMS/Thermomanagementsystem/Fluid/Fluid_Komponente thermisch/Konduktion 1. finites Volumen mit vorherigen Fluid_Komponenten - Vereinigung ==
  note: PQ_FinitesVolumen_FinitesVolumen_1 = (T_FinitesVolumen_vor1_n - T_FinitesVolumen_1) / R_Ersatz_1 + (T_FinitesVolumen_vor2_n - T_FinitesVolumen_1) / R_Ersatz_2
      | = Konduktion für das 1. finite Volumen mit vorherigen finiten Volumen
      |
      | mit R_Ersatz_1 = R_FinitesVolumen / (2 * 0.5) + R_FinitesVolumen_vor1 / 2 = R_FinitesVolumen + R_FinitesVolumen_vor1 / 2
      | mit R_Ersatz_2 = R_FinitesVolumen / (2 * 0.5) + R_FinitesVolumen_vor1 / 2 = R_FinitesVolumen + R_FinitesVolumen_vor2 / 2
      |
      | -> Dieses Subsystem repäsentiert den Fall, dass sich diese Fluid_Komponente nach der Vereinigung der zwei nach der Aufzweigung durch ein Dreiwegeventil resultierenden Pfade befindet
      | -> Diese Fluid_Komponente befindet sich nach 2 Fluid_Komponenten
      | -> Vor dieser Fluid_Komponente befindet sich kein Dreiwegeventil mit einem bestimmten Zustand, sondern es gilt die Annahme: Diese Fluid_Komponente steht mit 50% ihrer Querschnittsfläche der Kühlflüssigkeit in Beziehung mit Fluid_Komponente_vor1 und mit 50% ihrer Querschnittsfläche der Kühlflüssigkeit in Beziehung mit Fluid_Komponente_vor2
      |
      | -> Für die Herleitung dieses mathematischen Zusammenhangs wird auf die auf die im Rahmen des Thermomanagementsystemmodells erstellte Masterarbeit "Entwicklung und Steuerung eines Thermomanagementsystemmodells für Elektrofahrzeuge" verwiesen
  T_FinitesVolumen [K] : Inport
  R_FinitesVolumen [K*W^-1] : Inport  Port=2
  T_FinitesVolumen_vor1 [K] : Inport  Port=3
  R_FinitesVolumen_vor1 [K*W^-1] : Inport  Port=4
  T_FinitesVolumen_vor2 [K] : Inport  Port=5
  R_FinitesVolumen_vor2 [K*W^-1] : Inport  Port=6
  Add : Sum
  Add1 : Sum
  Gain : Gain  Gain=0.5
  Gain1 : Gain  Gain=0.5
  MATLAB Function : MATLAB Function  TreatAsAtomicUnit=on
  PQ_FinitesVolumen_FinitesVolumen [W] : Outport
  wires:
  T_FinitesVolumen [K]/1 -> MATLAB Function/1(u)
  MATLAB Function/1(y) -> PQ_FinitesVolumen_FinitesVolumen [W]/1
  R_FinitesVolumen_vor1 [K*W^-1]/1 -> Gain/1
  T_FinitesVolumen_vor1 [K]/1 -> MATLAB Function/2(v)
  R_FinitesVolumen_vor2 [K*W^-1]/1 -> Gain1/1
  T_FinitesVolumen_vor2 [K]/1 -> MATLAB Function/3(w)
  R_FinitesVolumen [K*W^-1]/1 -> Add/2, Add1/1
  Gain1/1 -> Add1/2
  Gain/1 -> Add/1
  Add/1 -> MATLAB Function/4(a)
  Add1/1 -> MATLAB Function/5(b)
